simulink model "GPSModel"  (Simulink 8.9)
settings: Solver=ode45  StartTime=0.0  StopTime=1000  RelTol=1e-3  EnableMultiTasking=on
values from neighbouring files (symbols this model uses):
  Height = [22.5395131711 22.5395131711 22.5395131711 16.5395131711 16.5395131711 16.5395131711 16.5395131711 16.5395131711 19.5395131711 19.5395131711 19.5395131711 19.5395131711 ... (2996 elements, 2996x1)]    [GPS.mat]    (also in GPS_database.m = Height - mean(Height))
  HeightX = (1:(1/Data_rate_Height):(LeHeight+Data_rate_Height-1)*(1/Data_rate_Height))'    [GPS_database.m]
  Latitude = [-4.47600000352 5.52399999648 10.5239999965 3.52399999648 20.5239999965 20.5239999965 32.5239999965 35.5239999965 33.5239999965 18.5239999965 18.5239999965 20.5239999965 ... (250 elements, 250x1)]    [GPS.mat]    (also in GPS_database.m = Latitude - mean(Latitude))
  LatitudeX = (1:(1/Data_rate_Latitude):(LeLat+Data_rate_Latitude-1)*(1/Data_rate_Latitude))'    [GPS_database.m]
  Longitude = [37.5840000007 37.5840000007 26.5840000007 21.5840000007 24.5840000007 27.5840000007 27.5840000007 21.5840000007 19.5840000007 16.5840000007 16.5840000007 16.5840000007 ... (250 elements, 250x1)]    [GPS.mat]    (also in GPS_database.m = Longitude - mean(Longitude))
  LongitudeX = (1:(1/Data_rate_Longitude):(LeLong+Data_rate_Longitude-1)*(1/Data_rate_Longitude))'    [GPS_database.m]
  TimeHe = ceil((LeHeight+3)*(1/Data_rate_Height))    [GPS_database.m]
  TimeLa = ceil((LeLat+Data_rate_Latitude-1)*(1/Data_rate_Latitude))    [GPS_database.m]
  TimeLo = ceil((LeLong+Data_rate_Longitude-1)*(1/Data_rate_Longitude))    [GPS_database.m]
settings Model: SuppressorTable=22 serialization::archive 11 0 6 0 0 0 11 0  Creator=Pau Kah Ho  LastModifiedBy=veikas
settings DataIOCC: SignalLoggingSaveFormat=Dataset
settings OptimizationCC: ExpressionDepthLimit=2147483647
settings DebuggingCC: SolverPrmCheckMsg=warning

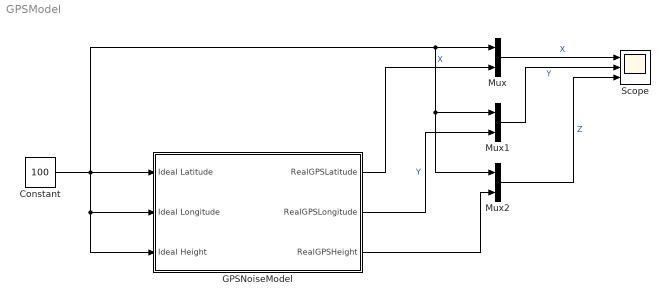
== system GPSModel ==
  Constant : Constant  Value=100
  GPSNoiseModel : Subsystem
  Mux : Mux  Inputs=2
  Mux1 : Mux  Inputs=2
  Mux2 : Mux  Inputs=2
  Scope : Scope  NumInputPorts=3
  wires:
  Constant/1 -> GPSNoiseModel/1(Ideal Latitude), GPSNoiseModel/2(Ideal Longitude), GPSNoiseModel/3(Ideal Height), Mux/1, Mux1/1, Mux2/1
  Mux/1 -> Scope/1  "X"
  Mux1/1 -> Scope/2  "Y"
  GPSNoiseModel/1(RealGPSLatitude) -> Mux/2  "X"
  GPSNoiseModel/2(RealGPSLongitude) -> Mux1/2  "Y"
  GPSNoiseModel/3(RealGPSHeight) -> Mux2/2
  Mux2/1 -> Scope/3  "Z"

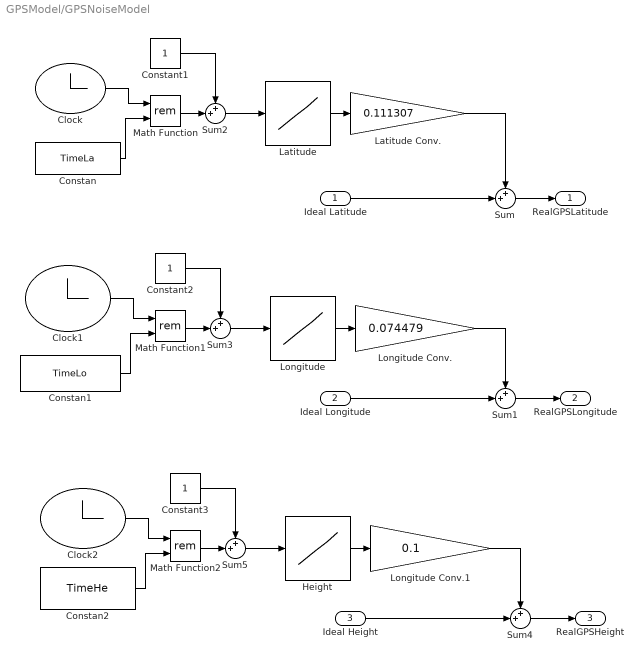
== system GPSModel/GPSNoiseModel ==
  Ideal Latitude : Inport
  Ideal Longitude : Inport  Port=2
  Ideal Height : Inport  Port=3
  Clock : Clock
  Clock1 : Clock
  Clock2 : Clock
  Constan : Constant  Value=TimeLa
  Constan1 : Constant  Value=TimeLo
  Constan2 : Constant  Value=TimeHe
  Constant1 : Constant
  Constant2 : Constant
  Constant3 : Constant
  Height : Lookup_n-D  NumberOfTableDimensions=1  BreakpointsForDimension1=HeightX  BreakpointsForDimension2=[1:3]  Table=Height  RndMeth=Simplest  InputSameDT=on
  Latitude : Lookup_n-D  NumberOfTableDimensions=1  BreakpointsForDimension1=LatitudeX  BreakpointsForDimension2=[1:3]  Table=Latitude  RndMeth=Simplest  InputSameDT=on
  Latitude Conv. : Gain  Gain=0.111307
  Longitude : Lookup_n-D  NumberOfTableDimensions=1  BreakpointsForDimension1=LongitudeX  BreakpointsForDimension2=[1:3]  Table=Longitude  RndMeth=Simplest  InputSameDT=on
  Longitude Conv. : Gain  Gain=0.074479
  Longitude Conv.1 : Gain  Gain=0.1
  Math Function : Math  Operator=rem  SaturateOnIntegerOverflow=on
  Math Function1 : Math  Operator=rem  SaturateOnIntegerOverflow=on
  Math Function2 : Math  Operator=rem  SaturateOnIntegerOverflow=on
  Sum{,1..5} (6 alike) : Sum  Inputs=++|
  RealGPSLatitude : Outport
  RealGPSLongitude : Outport  Port=2
  RealGPSHeight : Outport  Port=3
  wires:
  Latitude/1 -> Latitude Conv./1
  Ideal Latitude/1 -> Sum/2
  Ideal Longitude/1 -> Sum1/2
  Longitude/1 -> Longitude Conv./1
  Sum/1 -> RealGPSLatitude/1
  Sum1/1 -> RealGPSLongitude/1
  Latitude Conv./1 -> Sum/1
  Longitude Conv./1 -> Sum1/1
  Clock/1 -> Math Function/1
  Constan/1 -> Math Function/2
  Math Function/1 -> Sum2/2
  Constant1/1 -> Sum2/1
  Sum2/1 -> Latitude/1
  Clock1/1 -> Math Function1/1
  Constan1/1 -> Math Function1/2
  Math Function1/1 -> Sum3/2
  Constant2/1 -> Sum3/1
  Sum3/1 -> Longitude/1
  Ideal Height/1 -> Sum4/2
  Height/1 -> Longitude Conv.1/1
  Sum4/1 -> RealGPSHeight/1
  Longitude Conv.1/1 -> Sum4/1
  Clock2/1 -> Math Function2/1
  Constan2/1 -> Math Function2/2
  Math Function2/1 -> Sum5/2
  Constant3/1 -> Sum5/1
  Sum5/1 -> Height/1
